simulink subsystem "YawSubsystem"  (R2023b)
settings: Solver=VariableStepAuto  StartTime=0.0  StopTime=10.0  RelTol=1e-3
values from neighbouring files (symbols this model uses):
  Ixx = 15.67*10^(-3)    (= 0.01567)    [drone_input_params.m]
  Iyy = 15.67*10^(-3)    (= 0.01567)    [drone_input_params.m]
  Izz = 28.346*10^(-3)    (= 0.028346)    [drone_input_params.m]
settings Model: Creator=FRESH  LastModifiedBy=FRESH

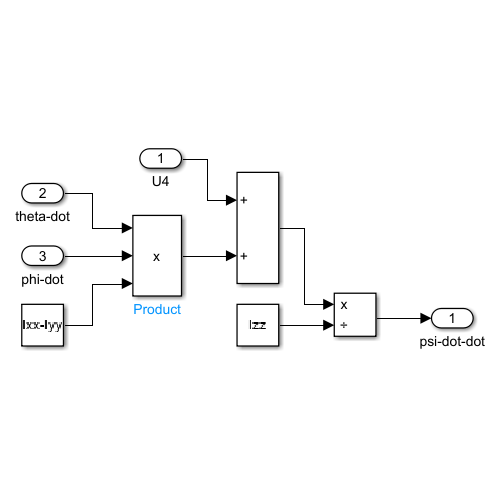
[thumbnail: Simulink's stored preview of the top-level diagram]
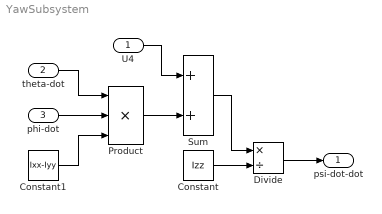
== system YawSubsystem ==
  U4 : Inport
  theta-dot : Inport  Port=2
  phi-dot : Inport  Port=3
  Constant : Constant  Value=Izz
  Constant1 : Constant  Value=Ixx-Iyy
  Divide : Product  Inputs=*/
  Product : Product  Inputs=3
  Sum : Sum
  psi-dot-dot : Outport
  wires:
  Divide/1 -> psi-dot-dot/1
  Sum/1 -> Divide/1
  theta-dot/1 -> Product/1
  phi-dot/1 -> Product/2
  Product/1 -> Sum/2
  Constant1/1 -> Product/3
  Constant/1 -> Divide/2
  U4/1 -> Sum/1
